simulink model "pokus_1"  (Simulink 8.0)
settings: Solver=ode1  SolverMode=SingleTasking  StartTime=0.0  StopTime=2.0  FixedStep=0.001  RelTol=1e-3
PostLoadFcn:
  | run('parametri.m');
values from neighbouring files (symbols this model uses):
  Beq = 4e-3    (= 0.004)    [parametri.m]
  Eff_G = 0.9    [parametri.m]
  Eff_M = 0.69    [parametri.m]
  Jeq = 2e-3    (= 0.002)    [parametri.m]
  Ke = 0.0076776    [parametri.m]
  Kg = 70    [parametri.m]
  Km = 0.007683    [parametri.m]
  Kp = omega^2*T/K    (= 29.3398872208)    [parametri.m]
  Kv = (2*zeta*omega*T-1)/K    (= 0.364280264132)    [parametri.m]
  Ra = 2.6    [parametri.m]
settings Model: Creator=Niko  LastModifiedBy=Niko

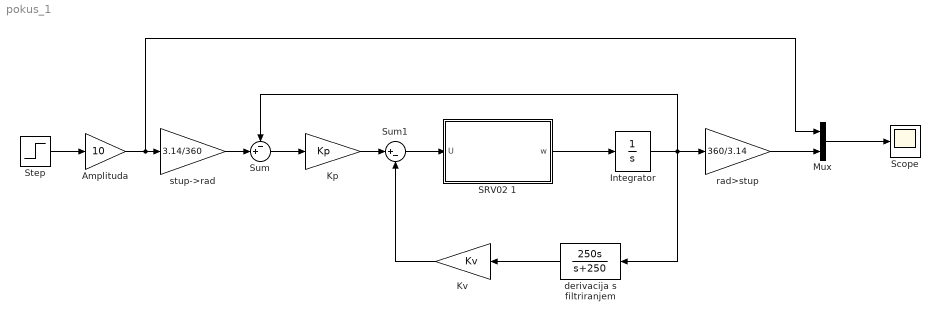
== system pokus_1 ==
  " derivacija s filtriranjem" : TransferFcn  Numerator=[250 0]  Denominator=[1 250]
  Amplituda : Gain  Gain=10
  Integrator : Integrator
  Kp : Gain  Gain=Kp
  Kv : Gain  Gain=Kv
  Mux : Mux  Inputs=2
  SRV02 1 : Subsystem
  Scope : Scope
      settings: TimeRange=5  YMin=0  YMax=30  SaveName=Response  SampleInput=on
  Step : Step  SampleTime=0
  Sum : Sum  Inputs=-+|
  Sum1 : Sum  Inputs=|+-
  rad>stup : Gain  Gain=360/3.14
  stup->rad : Gain  Gain=3.14/360
  wires:
  Integrator/1 -> rad>stup/1, Sum/1, " derivacija s filtriranjem"/1
  Kp/1 -> Sum1/1
  Sum/1 -> Kp/1
  " derivacija s filtriranjem"/1 -> Kv/1
  Kv/1 -> Sum1/2
  Sum1/1 -> SRV02 1/1(U)
  SRV02 1/1(w) -> Integrator/1
  Step/1 -> Amplituda/1
  stup->rad/1 -> Sum/2
  Amplituda/1 -> Mux/1, stup->rad/1
  rad>stup/1 -> Mux/2
  Mux/1 -> Scope/1

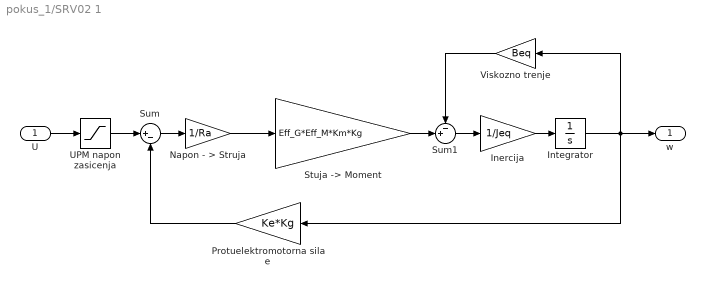
== system pokus_1/SRV02 1 ==
  U : Inport
  Inercija : Gain  Gain=1/Jeq
  Integrator : Integrator
  Napon - > Struja : Gain  Gain=1/Ra
  Protuelektromotorna sila e : Gain  Gain=Ke*Kg
  "Stuja -> Moment" : Gain  Gain=Eff_G*Eff_M*Km*Kg
  Sum : Sum  Inputs=|+-
  Sum1 : Sum  Inputs=-+|
  UPM napon zasicenja : Saturate  UpperLimit=6  LowerLimit=-6
  Viskozno trenje : Gain  Gain=Beq
  w : Outport
  wires:
  Sum1/1 -> Inercija/1
  "Stuja -> Moment"/1 -> Sum1/2
  Inercija/1 -> Integrator/1
  UPM napon zasicenja/1 -> Sum/1
  Napon - > Struja/1 -> "Stuja -> Moment"/1
  U/1 -> UPM napon zasicenja/1
  Sum/1 -> Napon - > Struja/1
  Viskozno trenje/1 -> Sum1/1
  Protuelektromotorna sila e/1 -> Sum/2
  Integrator/1 -> w/1, Protuelektromotorna sila e/1, Viskozno trenje/1
